simulink model "colas_PI"  (Simulink 2.09)
settings: Solver=ode15s  StartTime=0.0  StopTime=200  MaxStep=5  RelTol=1e-6  AbsTol=1e-6
settings Model: SaveTime=off  SaveOutput=off  ConsistencyChecking=off  RTWTemplateMakefile=grt_unix.tmf

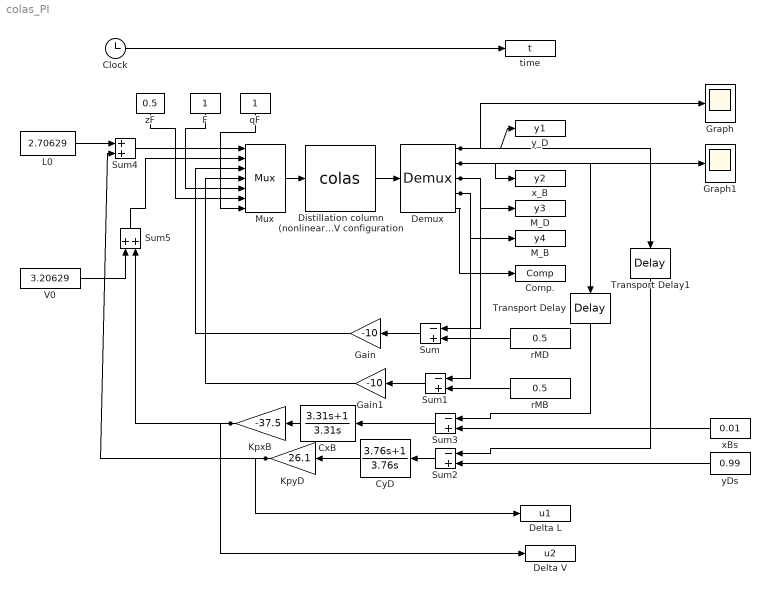
== system colas_PI ==
  " CyD" : TransferFcn  Orientation=left  Numerator=[3.76 1]  Denominator=[3.76 0]
  Clock : Clock
  Comp. : ToWorkspace  VariableName=Comp  SampleTime=0
      settings: Buffer=1200
  CxB : TransferFcn  Orientation=left  Numerator=[3.31 1]  Denominator=[3.31 0]
  Delta L : ToWorkspace  VariableName=u1  SampleTime=0
      settings: Buffer=1200
  Delta V : ToWorkspace  VariableName=u2  SampleTime=0
      settings: Buffer=1200
  Demux : Demux  Outputs=[1,1,1,1,41]
  Distillation column (nonlinear)  LV configuration : S-Function  FunctionName=colas
  F : Constant  Orientation=down  Value=1
  Gain : Gain  Orientation=left  Gain=-10
  Gain1 : Gain  Orientation=left  Gain=-10
  Graph : Scope
      settings: TickLabels=on  TimeRange=20  YMin=0.985  YMax=1  SaveToWorkspace=off  SaveName=ScopeData
  Graph1 : Scope
      settings: TickLabels=on  TimeRange=20  YMin=0  YMax=0.02  SaveToWorkspace=off  SaveName=ScopeData
  KpxB : Gain  Orientation=left  Gain=-37.5
  KpyD : Gain  Orientation=left  Gain=26.1
  L0 : Constant  Value=2.70629
  M_B : ToWorkspace  VariableName=y4  SampleTime=0
      settings: Buffer=1200
  M_D : ToWorkspace  VariableName=y3  SampleTime=0
      settings: Buffer=1200
  Mux : Mux  Inputs=7
  Sum{,1..3} (4 alike) : Sum  Orientation=left  Inputs=-+
  Sum4 : Sum  Inputs=++
  Sum5 : Sum  Orientation=up  Inputs=++
  Transport Delay : TransportDelay  Orientation=down  DelayTime=1  InitialInput=0.01  BufferSize=1024
  Transport Delay1 : TransportDelay  Orientation=down  DelayTime=1  InitialInput=0.99  BufferSize=1024
  V0 : Constant  Value=3.20629
  qF : Constant  Orientation=down  Value=1
  rMB : Constant  Orientation=left  Value=0.5
  rMD : Constant  Orientation=left  Value=0.5
  time : ToWorkspace  VariableName=t  SampleTime=0
      settings: Buffer=1000
  xBs : Constant  Orientation=left  Value=0.01
  x_B : ToWorkspace  VariableName=y2  SampleTime=0
      settings: Buffer=1200
  yDs : Constant  Orientation=left  Value=0.99
  y_D : ToWorkspace  VariableName=y1  SampleTime=0
      settings: Buffer=1200
  zF : Constant  Orientation=down  Value=0.5
  wires:
  yDs/1 -> Sum2/2
  xBs/1 -> Sum3/2
  Transport Delay1/1 -> Sum2/1
  Transport Delay/1 -> Sum3/1
  Demux/2 -> Transport Delay/1, Graph1/1, x_B/1
  KpxB/1 -> Delta V/1, Sum5/2
  KpyD/1 -> Delta L/1, Sum4/2
  " CyD"/1 -> KpyD/1
  CxB/1 -> KpxB/1
  Sum3/1 -> CxB/1
  Sum5/1 -> Mux/2
  V0/1 -> Sum5/1
  L0/1 -> Sum4/1
  Sum4/1 -> Mux/1
  Demux/1 -> Transport Delay1/1, Graph/1, y_D/1
  Sum2/1 -> " CyD"/1
  qF/1 -> Mux/7
  Gain1/1 -> Mux/4
  Sum1/1 -> Gain1/1
  rMB/1 -> Sum1/2
  Demux/4 -> Sum1/1, M_B/1
  Demux/3 -> Sum/1, M_D/1
  Gain/1 -> Mux/3
  rMD/1 -> Sum/2
  Sum/1 -> Gain/1
  Mux/1 -> Distillation column (nonlinear)  LV configuration/1
  Distillation column (nonlinear)  LV configuration/1 -> Demux/1
  Clock/1 -> time/1
  zF/1 -> Mux/6
  F/1 -> Mux/5
  Demux/5 -> Comp./1
